simulink subsystem "hor_vel_control"  (R2021a)
settings: Solver=VariableStepAuto  StartTime=0.0  StopTime=10.0  RelTol=1e-3
undefined symbols (not defined in the file or in its folder): C_vel, DiscIntNeverNeededParam
settings Model: Creator=EpEp  LastModifiedBy=EpEp

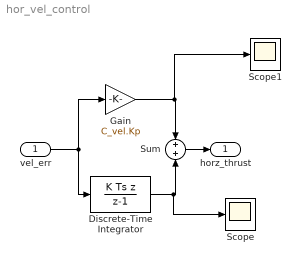
== system hor_vel_control ==
  vel_err : Inport
  Discrete-Time Integrator : DiscreteIntegrator  IntegratorMethod=Integration: Backward Euler  gainval=C_vel.Ki  SampleTime=C_vel.Ts  LimitOutput=on  UpperSaturationLimit=50  LowerSaturationLimit=-50  ICPrevOutput=DiscIntNeverNeededParam  ICPrevScaledInput=DiscIntNeverNeededParam
  Gain : Gain  Gain=C_vel.Kp
  Scope : Scope
  Scope1 : Scope
  Sum : Sum
  horz_thrust : Outport
  wires:
  vel_err/1 -> Gain/1, Discrete-Time Integrator/1
  Sum/1 -> horz_thrust/1
  Gain/1 -> Sum/1, Scope1/1
  Discrete-Time Integrator/1 -> Sum/2, Scope/1
